simulink model "busselector_test"  (Simulink 8.4)
settings: Solver=VariableStepDiscrete  StartTime=0.0  StopTime=0  MaxStep=1  RelTol=1e-3
settings Model: Creator=arnaud  LastModifiedBy=arnaud
settings DataIOCC: SaveFormat=Structure  SignalLoggingSaveFormat=Dataset
settings OptimizationCC: ExpressionDepthLimit=128
settings DebuggingCC: UnderspecifiedInitializationDetection=Simplified  MergeDetectMultiDrivingBlocksExec=error  FcnCallInpInsideContextMsg=EnableAllAsError  StateNameClashWarn=none
settings GRTTargetCC: CombineOutputUpdateFcns=on  GRTInterface=off

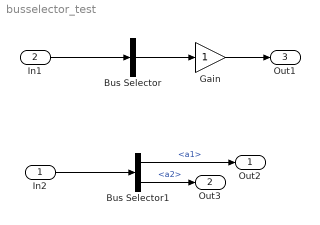
== system busselector_test ==
  In2 : Inport  OutDataTypeStr=Bus: BusA  BusOutputAsStruct=on
  In1 : Inport  Port=2  OutDataTypeStr=Bus: BusA
  Bus Selector : BusSelector  OutputSignals=a,a3  OutputAsBus=on
  Bus Selector1 : BusSelector  OutputSignals=a1,a2
  Gain : Gain
  Out2 : Outport
  Out3 : Outport  Port=2
  Out1 : Outport  Port=3
  wires:
  In2/1 -> Bus Selector1/1
  Bus Selector1/1 -> Out2/1  "<a1>"
  Bus Selector1/2 -> Out3/1  "<a2>"
  In1/1 -> Bus Selector/1
  Bus Selector/1 -> Gain/1
  Gain/1 -> Out1/1
